simulink model "AngleToPWM"  (R2014a)
settings: Solver=ode45  StartTime=0.0  StopTime=50000  RelTol=1e-3
libraries: hdlsllib x4, simulink x2
settings Model: Creator=scherb.a  LastModifiedBy=scherb.a
settings OptimizationCC: BlockReduction=off  ConditionallyExecuteInputs=off  InlineParams=on
settings DebuggingCC: AlgebraicLoopMsg=error
settings HardwareCC: ProdHWDeviceType=ASIC/FPGA->ASIC/FPGA  ProdEqTarget=off

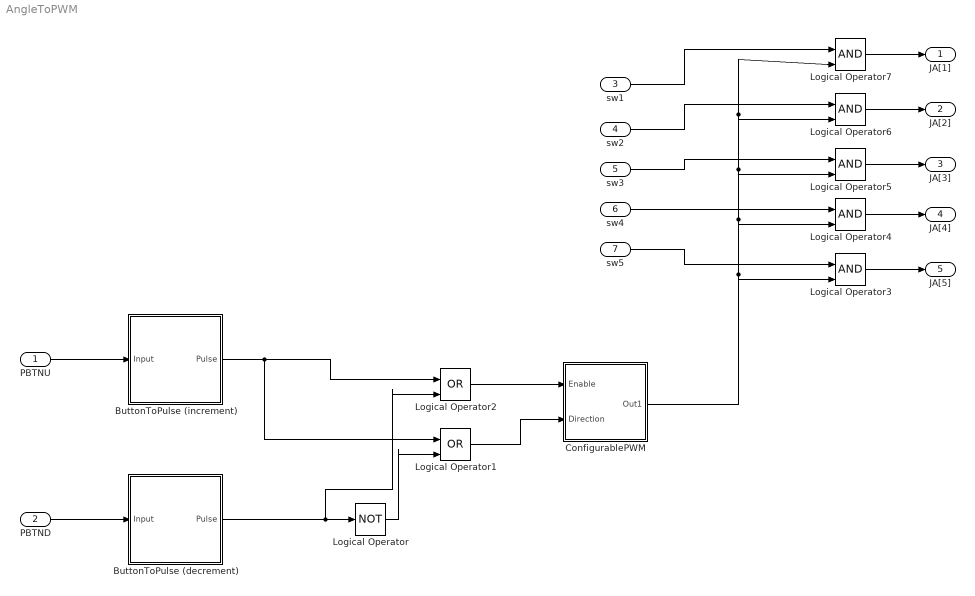
== system AngleToPWM ==
  PBTNU : Inport
  PBTND : Inport  Port=2
  sw1 : Inport  Port=3
  sw2 : Inport  Port=4
  sw3 : Inport  Port=5
  sw4 : Inport  Port=6
  sw5 : Inport  Port=7
  ButtonToPulse (decrement) : Subsystem
  ButtonToPulse (increment) : Subsystem
  ConfigurablePWM : Subsystem
  Logical Operator : Logic  Operator=NOT  IconShape=distinctive  AllPortsSameDT=off  OutDataTypeStr=boolean
  Logical Operator1 : Logic  Operator=OR  IconShape=distinctive  AllPortsSameDT=off  OutDataTypeStr=boolean
  Logical Operator2 : Logic  Operator=OR  IconShape=distinctive  AllPortsSameDT=off  OutDataTypeStr=boolean
  Logical Operator{3..7} (5 alike) : Logic  IconShape=distinctive  AllPortsSameDT=off  OutDataTypeStr=boolean
  JA[1] : Outport
  JA[2] : Outport  Port=2
  JA[3] : Outport  Port=3
  JA[4] : Outport  Port=4
  JA[5] : Outport  Port=5
  wires:
  Logical Operator2/1 -> ConfigurablePWM/1(Enable)
  Logical Operator1/1 -> ConfigurablePWM/2(Direction)
  Logical Operator/1 -> Logical Operator1/2
  ButtonToPulse (decrement)/1(Pulse) -> Logical Operator2/2, Logical Operator/1
  ButtonToPulse (increment)/1(Pulse) -> Logical Operator1/1, Logical Operator2/1
  PBTNU/1 -> ButtonToPulse (increment)/1(Input)
  PBTND/1 -> ButtonToPulse (decrement)/1(Input)
  Logical Operator4/1 -> JA[4]/1
  Logical Operator3/1 -> JA[5]/1
  Logical Operator5/1 -> JA[3]/1
  Logical Operator6/1 -> JA[2]/1
  Logical Operator7/1 -> JA[1]/1
  ConfigurablePWM/1(Out1) -> Logical Operator7/2, Logical Operator6/2, Logical Operator5/2, Logical Operator4/2, Logical Operator3/2
  sw1/1 -> Logical Operator7/1
  sw2/1 -> Logical Operator6/1
  sw3/1 -> Logical Operator5/1
  sw4/1 -> Logical Operator4/1
  sw5/1 -> Logical Operator3/1

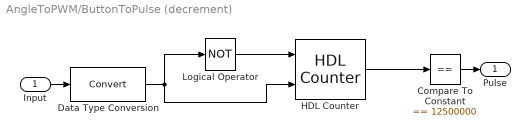
== system AngleToPWM/ButtonToPulse (decrement) ==
  Input : Inport
  Compare To Constant : simulink/Logic and Bit Operations/Compare To Constant  relop===  const=12500000  OutDataTypeStr=boolean
  Data Type Conversion : DataTypeConversion
  HDL Counter : hdlsllib/HDL Operations/HDL Counter  CountType=Count limited  CountInit=0  CountStep=1  CountMax=50000000  CountFromType=Initial value  CountFrom=0  CountResetPort=on  CountLoadPort=off  CountEnbPort=on  CountDirPort=off  CountDataType=Unsigned  CountWordLen=32  CountFracLen=0  CountSampTime=1
  Logical Operator : Logic  Operator=NOT  IconShape=distinctive  AllPortsSameDT=off  OutDataTypeStr=boolean
  Pulse : Outport
  wires:
  HDL Counter/1 -> Compare To Constant/1
  Logical Operator/1 -> HDL Counter/1
  Data Type Conversion/1 -> HDL Counter/2, Logical Operator/1
  Compare To Constant/1 -> Pulse/1
  Input/1 -> Data Type Conversion/1

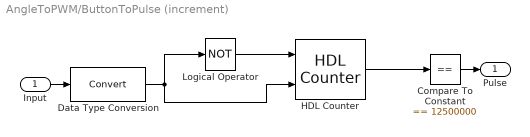
== system AngleToPWM/ButtonToPulse (increment) ==
  Input : Inport
  Compare To Constant : simulink/Logic and Bit Operations/Compare To Constant  relop===  const=12500000  OutDataTypeStr=boolean
  Data Type Conversion : DataTypeConversion
  HDL Counter : hdlsllib/HDL Operations/HDL Counter  CountType=Count limited  CountInit=0  CountStep=1  CountMax=50000000  CountFromType=Initial value  CountFrom=0  CountResetPort=on  CountLoadPort=off  CountEnbPort=on  CountDirPort=off  CountDataType=Unsigned  CountWordLen=32  CountFracLen=0  CountSampTime=1
  Logical Operator : Logic  Operator=NOT  IconShape=distinctive  AllPortsSameDT=off  OutDataTypeStr=boolean
  Pulse : Outport
  wires:
  HDL Counter/1 -> Compare To Constant/1
  Logical Operator/1 -> HDL Counter/1
  Data Type Conversion/1 -> HDL Counter/2, Logical Operator/1
  Compare To Constant/1 -> Pulse/1
  Input/1 -> Data Type Conversion/1

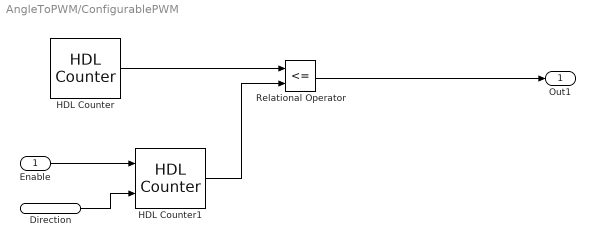
== system AngleToPWM/ConfigurablePWM ==
  Enable : Inport
  Direction : Inport  Port=2
  HDL Counter : hdlsllib/HDL Operations/HDL Counter  CountType=Count limited  CountInit=0  CountStep=1  CountMax=1000000  CountFromType=Initial value  CountFrom=0  CountResetPort=off  CountLoadPort=off  CountEnbPort=off  CountDirPort=off  CountDataType=Unsigned  CountWordLen=20  CountFracLen=0  CountSampTime=1
  HDL Counter1 : hdlsllib/HDL Operations/HDL Counter  CountType=Count limited  CountInit=75000  CountStep=6000  CountMax=120000  CountFromType=Specify  CountFrom=30000  CountResetPort=off  CountLoadPort=off  CountEnbPort=on  CountDirPort=on  CountDataType=Unsigned  CountWordLen=32  CountFracLen=0  CountSampTime=1
  Relational Operator : RelationalOperator  Operator=<=  OutDataTypeStr=boolean
  Out1 : Outport
  wires:
  Enable/1 -> HDL Counter1/1
  HDL Counter1/1 -> Relational Operator/2
  Direction/1 -> HDL Counter1/2
  HDL Counter/1 -> Relational Operator/1
  Relational Operator/1 -> Out1/1
